simulink model "logo_monitoring_task"  (Simulink 3.00)
libraries: lib x4, mathlib x2

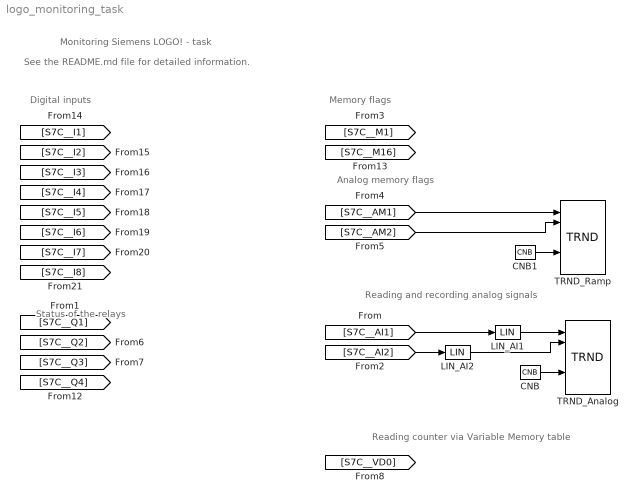
== system logo_monitoring_task ==
  note: Digital inputs
  note: Status of the relays
  note: Analog memory flags
  note: Memory flags
  note: Reading counter via Variable Memory table
  note: Reading and recording analog signals
  note: See the README.md file for detailed information.
  note: Monitoring Siemens LOGO! - task
  CNB : lib/CNB  YCN=on
  CNB1 : lib/CNB  YCN=on
  LIN_AI1 : mathlib/LIN  u1=0  y1=0  u2=1000  y2=10
  LIN_AI2 : mathlib/LIN  u1=0  y1=0  u2=1000  y2=10
  TRND_Analog : lib/TRND  n=2  l=9000  btype=8: Double  ptype1=1: Store  ptype2=1: Store  ptype3=1: Store  ptype4=1: Store  pfac=1  afac=0  arc=0  id=2  Title=Analog signals  timesrc=1
  TRND_Ramp : lib/TRND  n=2  l=9000  btype=8: Double  ptype1=1: Store  ptype2=1: Store  ptype3=1: Store  ptype4=1: Store  pfac=1  afac=0  arc=0  id=2  Title=Ramp signal and sample&hold  timesrc=1
  wires:
  CNB/1 -> TRND_Analog/5
  CNB1/1 -> TRND_Ramp/5
  [S7C__AI1] -> LIN_AI1/1
  [S7C__AI2] -> LIN_AI2/1
  [S7C__AM1] -> TRND_Ramp/1
  [S7C__AM2] -> TRND_Ramp/2
  LIN_AI1/1 -> TRND_Analog/1
  LIN_AI2/1 -> TRND_Analog/2
